simulink model "Demo_init"  (R2023a)
settings: Solver=ode23tb  StartTime=0.0  StopTime=630  RelTol=1e-3
undefined symbols (not defined in the file): i_gearbox_1, i_gearbox_2, J_gearbox_1, J_gearbox_2
settings Model: Creator=Maxim Kozlov  LastModifiedBy=ycheb

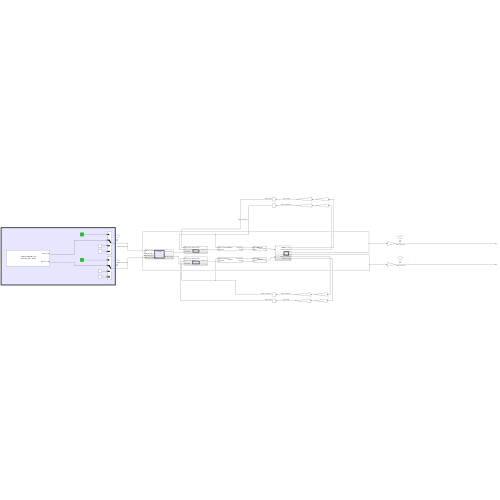
[thumbnail: Simulink's stored preview of the top-level diagram]
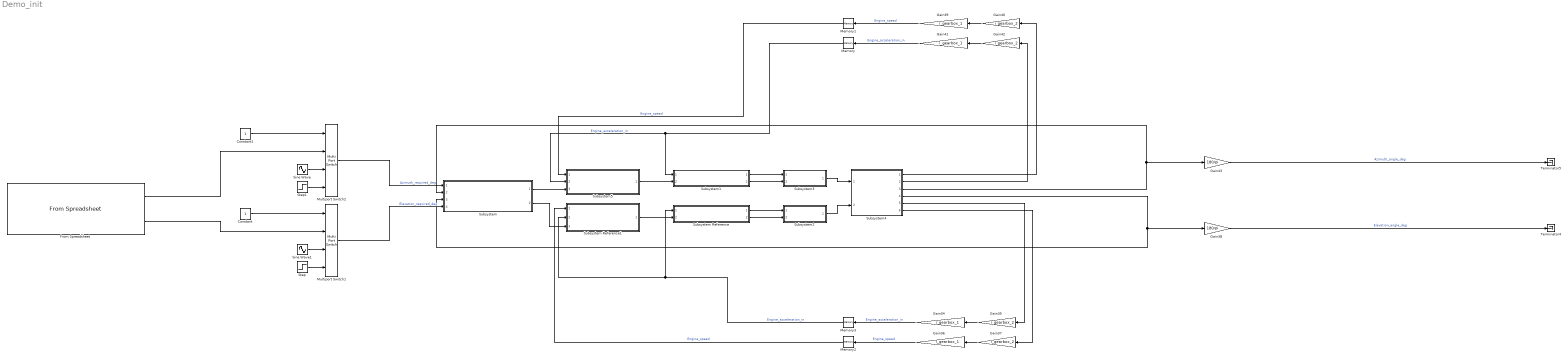
== system Demo_init ==
  Constant : Constant
  Constant1 : Constant
  From Spreadsheet : FromSpreadsheet  FileName=.\data\DemoSatelliteData.xlsx  SheetName=International_Space_Station
  Gain{34,36,39,41} (4 alike) : Gain  Gain=i_gearbox_1
  Gain{35,37,40,42} (4 alike) : Gain  Gain=i_gearbox_2
  Gain38 : Gain  Gain=180/pi
  Gain43 : Gain  Gain=180/pi
  Memory{,1..3} (4 alike) : Memory
  Multiport Switch1 : MultiPortSwitch  SaturateOnIntegerOverflow=off  InputSameDT=off
  Multiport Switch2 : MultiPortSwitch  SaturateOnIntegerOverflow=off  InputSameDT=off
  Sine Wave : Sin  Amplitude=6  Phase=pi/2  SampleTime=0
  Sine Wave1 : Sin  Amplitude=6  SampleTime=0
  Step : Step  SampleTime=0
  Step1 : Step  SampleTime=0
  Subsystem : Subsystem  ReferencedSubsystem=Converter
  Subsystem Reference : Subsystem  ReferencedSubsystem=Reductor  J=J_gearbox_1  i=i_gearbox_1
  Subsystem Reference1 : Subsystem  ReferencedSubsystem=Electric_motor
  Subsystem1 : Subsystem  ReferencedSubsystem=Reductor  J=J_gearbox_1  i=i_gearbox_1
  Subsystem2 : Subsystem  ReferencedSubsystem=Reductor2  J=J_gearbox_2  i=i_gearbox_2
  Subsystem3 : Subsystem  ReferencedSubsystem=Reductor2  J=J_gearbox_2  i=i_gearbox_2
  Subsystem4 : Subsystem  ReferencedSubsystem=Object
  Subsystem5 : Subsystem  ReferencedSubsystem=Electric_motor
  Terminator4 : Terminator
  Terminator5 : Terminator
  wires:
  Gain34/1 -> Memory3/1  "Engine_acceleration_in"
  Constant/1 -> Multiport Switch1/1
  Gain39/1 -> Memory1/1  "Engine_speed"
  Gain43/1 -> Terminator5/1  "Azimuth_angle_deg"
  Gain40/1 -> Gain39/1
  Gain42/1 -> Gain41/1
  Sine Wave1/1 -> Multiport Switch1/3
  Gain41/1 -> Memory/1  "Engine_acceleration_in"
  Gain36/1 -> Memory2/1  "Engine_speed"
  Gain37/1 -> Gain36/1
  Gain38/1 -> Terminator4/1  "Elevation_angle_deg"
  From Spreadsheet/1 -> Multiport Switch2/2
  From Spreadsheet/2 -> Multiport Switch1/2
  Step1/1 -> Multiport Switch2/4
  Constant1/1 -> Multiport Switch2/1
  Gain35/1 -> Gain34/1
  Sine Wave/1 -> Multiport Switch2/3
  Step/1 -> Multiport Switch1/4
  Memory/1 -> Subsystem5/2, Subsystem1/1  "Engine_acceleration_in"
  Multiport Switch2/1 -> Subsystem/1  "Azimuth_required_deg"
  Multiport Switch1/1 -> Subsystem/4  "Elevation_required_deg"
  Subsystem Reference/1 -> Subsystem2/1
  Subsystem Reference/2 -> Subsystem2/2
  Subsystem1/1 -> Subsystem3/1
  Subsystem1/2 -> Subsystem3/2
  Subsystem4/4 -> Gain38/1, Subsystem/3
  Subsystem4/3 -> Gain43/1, Subsystem/2
  Subsystem3/1 -> Subsystem4/1
  Subsystem2/1 -> Subsystem4/2
  Subsystem4/1 -> Gain40/1
  Subsystem4/2 -> Gain42/1
  Subsystem4/5 -> Gain35/1
  Subsystem4/6 -> Gain37/1
  Memory1/1 -> Subsystem5/1  "Engine_speed"
  Subsystem/1 -> Subsystem5/3
  Subsystem5/1 -> Subsystem1/2
  Subsystem Reference1/1 -> Subsystem Reference/2
  Memory3/1 -> Subsystem Reference/1, Subsystem Reference1/2  "Engine_acceleration_in"
  Memory2/1 -> Subsystem Reference1/1  "Engine_speed"
  Subsystem/2 -> Subsystem Reference1/3
